simulink model "demod_model_composer"  (R2021b)
settings: Solver=VariableStepAuto  StartTime=0.0  StopTime=20  RelTol=1e-3
undefined symbols (not defined in the file): A, N, xc7a35tiftg256
libraries: hlsBasic x32, dspvision x2, commanapbnd3 x1, hlsUtilities x1, hlsMath x1, vmcUtilities x1, simulink_extras x1
settings Model: Creator=caccolillo  LastModifiedBy=caccolillo

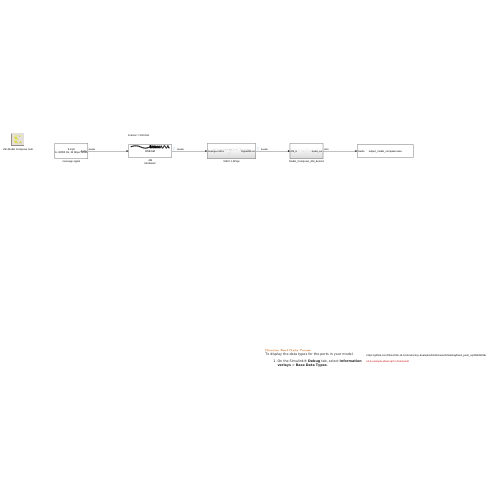
[thumbnail: Simulink's stored preview of the top-level diagram]
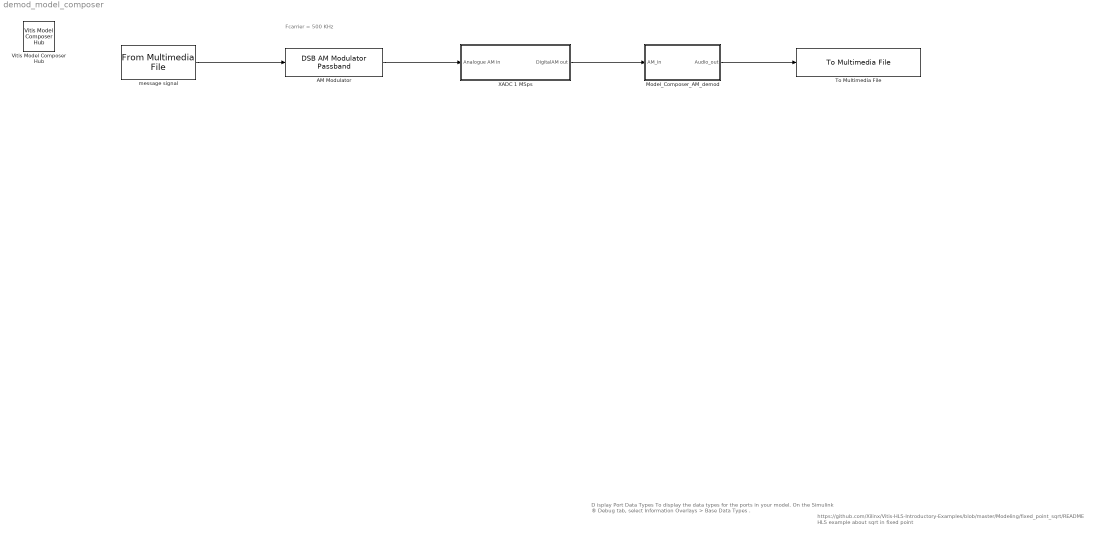
== system demod_model_composer ==
  note: https://github.com/Xilinx/Vitis-HLS-Introductory-Examples/blob/master/Modeling/fixed_point_sqrt/README
      |
      | HLS example about sqrt in fixed point
  note: D isplay Port Data Types
      | To display the data types for the ports in your model.
      | On the Simulink ® Debug tab, select Information Overlays > Base Data Types .
  note: Fcarrier = 500 KHz
  " AM Modulator " : commanapbnd3/DSB AM Modulator Passband  Fc=500000  Ph=0  Offset=1
      settings: SourceProductBaseCode=CM
  Model_Composer_AM_demod : Subsystem
  To Multimedia File : dspvision/To Multimedia File  outputFilename=output_model_composer.wav  streamSelection=Audio only  videoCompressor=None (uncompressed)  audioCompressor=None (uncompressed)  imagePorts=Separate color signals  fileType=WAV  audioDatatype=16-bit integer  fourcc=RGB  videoQuality=75  mj2000CompFactor=10
  Vitis Model Composer Hub : vmcUtilities/Vitis Model Composer Hub  Tag=genX  CodeGeneration=off  SubsystemName=Model_Composer_AM_demod  TargetDirectory=./code  ExportType=IP Catalog  IpVendor=xilinx.com  IpLibrary=hls  IpName=Model_Composer_AM_demod  IpVersion=1.0  IpHWLanguage=VHDL  AieCompilerOptions={}  CreateTestbench=off  TestbenchStackSize=10  RunAieSim=off  AieSimTimeout=50000  RunAieSimProfiling=off  LaunchVitisAnalyzer=off  PlotOutput=off  RunX86Sim=off  X86SimTimeout=10  GenHwImage=off  PlatformType=Not Specified  HwSystemType=Baremetal  HwValidationTarget=hw  ProjDevice=xc7a35tiftg256-1L  ProjDevicePart=xc7a35tiftg256-1L  SamplePeriod=-1  ClockFrequency=200  DataPathParallelism=1  xilinxfamily=artix7  part=xc7a35ti  speed=-1L  package=ftg256  directory=/home/caccolillo/Documents/model_composer_am_demod_v3/codegen  testbench=on  incr_netlist=off  synthesis_tool=Vivado  clock_wrapper=Clock Enables  dbl_ovrd=According to Block Masks  dcm_input_clock_period=10  sysclk_period=10  simulink_period=1/1e6  eval_field=0  IPInfoJsonString="{\"HLSSubsystem\":{\"SubsystemName\":\"Model_Composer_AM_demod\",\"IPName\":\"Model_Composer_AM_demod\",\"IPLibrary\":\"hls\",\"IPVendor\":\"xilinx.com\",\"IPVersion\":\"1.0\"}}"
  XADC 1 MSps : Subsystem
  message signal : dspvision/From Multimedia File  inputFilename=/home/caccolillo/Documents/model_composer_am_demod/audio/2.mp3  readRange=[1 Inf]  loop=on  numPlays=inf  outputStreams=Audio only  videoDataType=single  audioDataType=double  inheritSampleTime=on  userDefinedSampleTime=1/30  noAudioOutput=off  isIntensityVideo=off  fourcc=RGB  colorVideoFormat=Separate color signals  outputEOF=off  dataOrg=Column-major  audioFrameSize=1  computeAudioFrameSize=off  outSamplingMode=Frame based
  wires:
  " AM Modulator "/1 -> XADC 1 MSps/1(Analogue AM in)
  message signal/1 -> " AM Modulator "/1
  XADC 1 MSps/1(DigitalAM out) -> Model_Composer_AM_demod/1(AM_in)
  Model_Composer_AM_demod/1(Audio_out) -> To Multimedia File/1

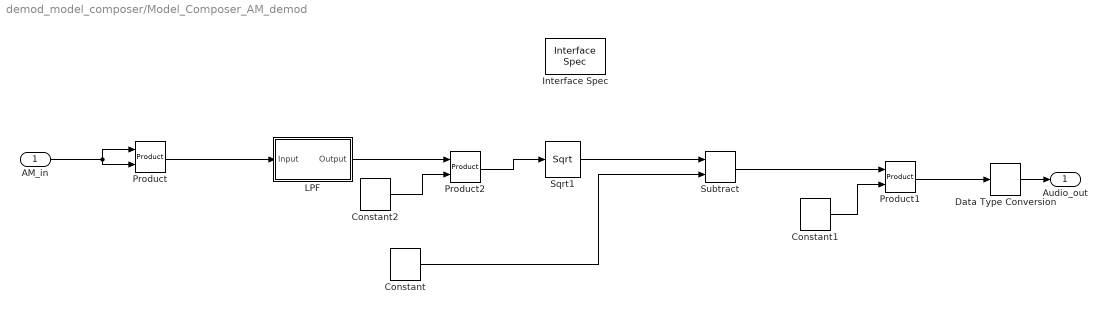
== system demod_model_composer/Model_Composer_AM_demod ==
  AM_in : Inport
  Constant : hlsBasic/Constant  Value=1365  SampleTime=-1  OutDataType=double  TypeExp=''  Signedness=Signed  WordLength=16  FractionalLength=0  RoundingMode=Truncation to minus infinity  OverflowMode=Wrap around
  Constant1 : hlsBasic/Constant  Value=2  SampleTime=-1  OutDataType=double  TypeExp=''  Signedness=Signed  WordLength=16  FractionalLength=0  RoundingMode=Truncation to minus infinity  OverflowMode=Wrap around
  Constant2 : hlsBasic/Constant  Value=2  SampleTime=-1  OutDataType=double  TypeExp=''  Signedness=Signed  WordLength=16  FractionalLength=0  RoundingMode=Truncation to minus infinity  OverflowMode=Wrap around
  Data Type Conversion : hlsBasic/Data Type Conversion  OutDataType=int16  TypeExp=''  Signedness=Signed  WordLength=16  FractionalLength=0  RoundingMode=Truncation to minus infinity  OverflowMode=Wrap around
  Interface Spec : hlsUtilities/Interface Spec  Return=AXI4-Lite Slave@@  InportInterfaces={'FIFO@@@N/A@N/A'}  InportHandles={3.730051269531250000e+02}  InportNames={'AM_in'}  OutportInterfaces={'FIFO@@@N/A@N/A'}  OutportHandles={4.820048828125000000e+02}  OutportNames={'Audio_out'}  Mode=AXI4-Lite Slave  InName1=AM_in  InMode1=FIFO  InVFormat1=N/A  InVComponent1=N/A  InMode2=Default  InVFormat2=N/A  InVComponent2=N/A  InMode3=Default  InVFormat3=N/A  InVComponent3=N/A  InMode4=Default  InVFormat4=N/A  InVComponent4=N/A  InMode5=Default  InVFormat5=N/A  InVComponent5=N/A  InMode6=Default  InVFormat6=N/A  InVComponent6=N/A  InMode7=Default  InVFormat7=N/A  InVComponent7=N/A  InMode8=Default  InVFormat8=N/A  InVComponent8=N/A  OutName1=Audio_out  OutMode1=FIFO  OutVFormat1=N/A  OutVComponent1=N/A  OutMode2=Default  OutVFormat2=N/A  OutVComponent2=N/A  OutMode3=Default  OutVFormat3=N/A  OutVComponent3=N/A  OutMode4=Default  OutVFormat4=N/A  OutVComponent4=N/A  OutMode5=Default  OutVFormat5=N/A  OutVComponent5=N/A  OutMode6=Default  OutVFormat6=N/A  OutVComponent6=N/A  OutMode7=Default  OutVFormat7=N/A  OutVComponent7=N/A  OutMode8=Default  OutVFormat8=N/A  OutVComponent8=N/A
  LPF : Subsystem  Tag=FilterWizardSubSystem
      settings: ErrorFcn=dspFilterRealizedInBasicElemsAlgLoopErrFcnCallback
  Product : hlsBasic/Product
  Product1 : hlsBasic/Product
  Product2 : hlsBasic/Product
  Sqrt1 : hlsMath/Sqrt
  Subtract : hlsBasic/Subtract
  Audio_out : Outport
  wires:
  Data Type Conversion/1 -> Audio_out/1
  Product1/1 -> Data Type Conversion/1
  Constant1/1 -> Product1/2
  Product2/1 -> Sqrt1/1
  Constant2/1 -> Product2/2
  Product/1 -> LPF/1(Input)
  AM_in/1 -> Product/2, Product/1
  LPF/1(Output) -> Product2/1
  Constant/1 -> Subtract/2
  Subtract/1 -> Product1/1
  Sqrt1/1 -> Subtract/1

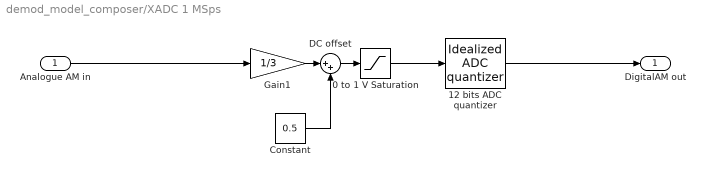
== system demod_model_composer/XADC 1 MSps ==
  Analogue AM in : Inport
  0 to 1 V Saturation : Saturate  UpperLimit=1  LowerLimit=0
  12 bits ADC quantizer : simulink_extras/Additional Discrete/Idealized ADC quantizer  NumberOfConverterBits=12  Vmin=0  Vmax=1  OutputDataType=double  OutputNegativeValues=on
  Constant : Constant  Value=0.5
  DC offset : Sum  Inputs=|++
  Gain1 : Gain  Gain=1/3
  DigitalAM out : Outport
  wires:
  DC offset/1 -> 0 to 1 V Saturation/1
  0 to 1 V Saturation/1 -> 12 bits ADC quantizer/1
  Constant/1 -> DC offset/2
  Gain1/1 -> DC offset/1
  12 bits ADC quantizer/1 -> DigitalAM out/1
  Analogue AM in/1 -> Gain1/1

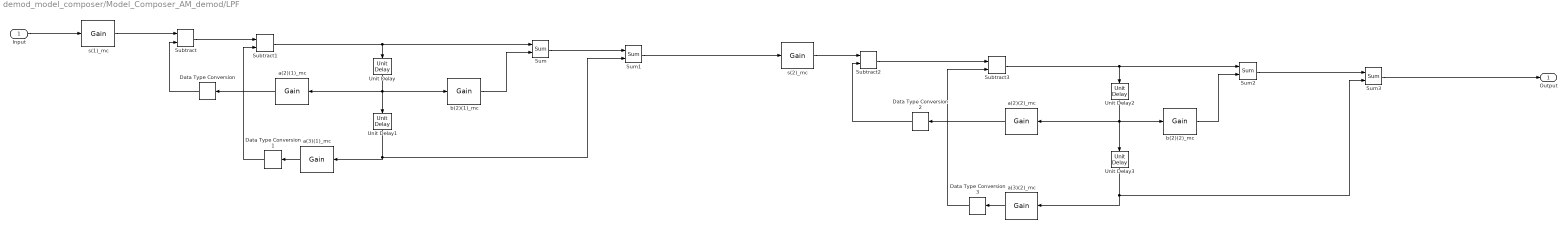
== system demod_model_composer/Model_Composer_AM_demod/LPF ==
  Input : Inport
  Data Type Conversion : hlsBasic/Data Type Conversion  OutDataType=fixed  TypeExp=''  Signedness=Signed  WordLength=67  FractionalLength=17  RoundingMode=Truncation to minus infinity  OverflowMode=Wrap around
  Data Type Conversion1 : hlsBasic/Data Type Conversion  OutDataType=fixed  TypeExp=''  Signedness=Signed  WordLength=68  FractionalLength=17  RoundingMode=Truncation to minus infinity  OverflowMode=Wrap around
  Data Type Conversion2 : hlsBasic/Data Type Conversion  OutDataType=fixed  TypeExp=''  Signedness=Signed  WordLength=157  FractionalLength=51  RoundingMode=Truncation to minus infinity  OverflowMode=Wrap around
  Data Type Conversion3 : hlsBasic/Data Type Conversion  OutDataType=fixed  TypeExp=''  Signedness=Signed  WordLength=158  FractionalLength=51  RoundingMode=Truncation to minus infinity  OverflowMode=Wrap around
  Subtract{,1..3} (4 alike) : hlsBasic/Subtract
  Sum{,1..3} (4 alike) : hlsBasic/Sum
  Unit Delay{,1..3} (4 alike) : hlsBasic/Unit Delay  InitialCondition=0
  a(2)(1)_mc : hlsBasic/Gain  Gain=-1.70096433194352592  OutDataType=fixed  TypeExp=''  Signedness=Signed  WordLength=69  FractionalLength=17  RoundingMode=Truncation to minus infinity  OverflowMode=Wrap around  OutputTypeAsInput=off
  a(2)(2)_mc : hlsBasic/Gain  Gain=-1.47967421693119339  OutDataType=fixed  TypeExp=''  Signedness=Signed  WordLength=43  FractionalLength=17  RoundingMode=Truncation to minus infinity  OverflowMode=Wrap around  OutputTypeAsInput=off
  a(3)(1)_mc : hlsBasic/Gain  Gain=0.788499739815297973  OutDataType=fixed  TypeExp=''  Signedness=Signed  WordLength=43  FractionalLength=17  RoundingMode=Truncation to minus infinity  OverflowMode=Wrap around  OutputTypeAsInput=off
  a(3)(2)_mc : hlsBasic/Gain  Gain=0.555821543282489006  OutDataType=fixed  TypeExp=''  Signedness=Signed  WordLength=43  FractionalLength=17  RoundingMode=Truncation to minus infinity  OverflowMode=Wrap around  OutputTypeAsInput=off
  b(2)(1)_mc : hlsBasic/Gain  Gain=2  OutDataType=fixed  TypeExp=''  Signedness=Signed  WordLength=43  FractionalLength=17  RoundingMode=Truncation to minus infinity  OverflowMode=Wrap around  OutputTypeAsInput=off
  b(2)(2)_mc : hlsBasic/Gain  Gain=2  OutDataType=fixed  TypeExp=''  Signedness=Signed  WordLength=43  FractionalLength=17  RoundingMode=Truncation to minus infinity  OverflowMode=Wrap around  OutputTypeAsInput=off
  s(1)_mc : hlsBasic/Gain  Gain=0.0218838519679430236  OutDataType=fixed  TypeExp=''  Signedness=Signed  WordLength=43  FractionalLength=17  RoundingMode=Truncation to minus infinity  OverflowMode=Wrap around  OutputTypeAsInput=off
  s(2)_mc : hlsBasic/Gain  Gain=0.0190368315878238735  OutDataType=fixed  TypeExp=''  Signedness=Signed  WordLength=43  FractionalLength=17  RoundingMode=Truncation to minus infinity  OverflowMode=Wrap around  OutputTypeAsInput=off
  Output : Outport
  wires:
  Input/1 -> s(1)_mc/1
  s(1)_mc/1 -> Subtract/1
  Subtract/1 -> Subtract1/1
  Subtract1/1 -> Sum/1, Unit Delay/1
  Unit Delay/1 -> b(2)(1)_mc/1, a(2)(1)_mc/1, Unit Delay1/1
  a(2)(1)_mc/1 -> Data Type Conversion/1
  Unit Delay1/1 -> Sum1/2, a(3)(1)_mc/1
  a(3)(1)_mc/1 -> Data Type Conversion1/1
  b(2)(1)_mc/1 -> Sum/2
  Sum/1 -> Sum1/1
  Sum1/1 -> s(2)_mc/1
  Subtract2/1 -> Subtract3/1
  s(2)_mc/1 -> Subtract2/1
  Subtract3/1 -> Sum2/1, Unit Delay2/1
  Unit Delay2/1 -> b(2)(2)_mc/1, Unit Delay3/1, a(2)(2)_mc/1
  Sum2/1 -> Sum3/1
  Sum3/1 -> Output/1
  a(2)(2)_mc/1 -> Data Type Conversion2/1
  a(3)(2)_mc/1 -> Data Type Conversion3/1
  b(2)(2)_mc/1 -> Sum2/2
  Unit Delay3/1 -> Sum3/2, a(3)(2)_mc/1
  Data Type Conversion/1 -> Subtract/2
  Data Type Conversion1/1 -> Subtract1/2
  Data Type Conversion2/1 -> Subtract2/2
  Data Type Conversion3/1 -> Subtract3/2
